simulink model "gm_uz_pmsm_model_9ph_21b_all_double"  (R2021b)
settings: Solver=FixedStepDiscrete  StartTime=0.0  StopTime=0.8  RelTol=1e-3
PreLoadFcn:
  | uz_pmsm_model_9ph_init_parameter
undefined symbols (not defined in the file or in its folder): a, b, c, friction_coefficient, inertia, k_i_d, k_i_q, k_p_d, k_p_q, Kpd, L_d, L_o1, L_o2, L_q, L_x1, L_x2, L_y1, L_y2, L_zero, polepair, psi_pm, R_1, static_friction_torque, Tnd
libraries: hdlmdlgenlib x139, hdlsllib x90, dspsigops x21, simulink x3, slpidlib x2, spsAlphaBetaZerotodq0Lib x1, pid_lib x1, spsdq0toAlphaBetaZeroLib x1
(part 4 of 5)

== system gm_uz_pmsm_model_9ph_21b_all_double/uz_pmsm_model_9ph/Line-Line to Phase voltage2/alpha_beta_0   to   abc ==
  "alpha, beta, 0  " : Inport  OutDataTypeStr=fixdt(1, 25, 12)  PortDimensions=[3]  SampleTime=1e-08
  Gain4_const : Constant  Value=[1;-0.5;-0.5;0;0.86602783203125;-0.86602783203125;1;1;1]  OutDataTypeStr=fixdt(1, 18, 16)  SampleTime=1e-08
  HwModeRegister : Delay  DelayLength=double(1)  InitialCondition=0  SampleTime=1e-08
  HwModeRegister1 : Delay  DelayLength=double(1)  InitialCondition=0  SampleTime=1e-08
  MMul_add_01 : Sum  OutDataTypeStr=fixdt(1, 25, 12)  SaturateOnIntegerOverflow=on  SampleTime=1e-08
  MMul_add_12 : Sum  OutDataTypeStr=fixdt(1, 25, 12)  SaturateOnIntegerOverflow=on  SampleTime=1e-08
  MMul_dot_product : Product  Inputs=**  OutDataTypeStr=fixdt(1, 43, 28)  SampleTime=1e-08
  MMul_dot_product_out_dtc : DataTypeConversion  OutDataTypeStr=fixdt(1, 25, 12)  SampleTime=1e-08  SaturateOnIntegerOverflow=on
  PipelineRegister : Delay  DelayLength=double(1)  InitialCondition=0  SampleTime=1e-08
  Reshape : Reshape  OutputDimensionality=Column vector (2-D)
  Row2Col_in0 : Reshape  OutputDimensionality=Column vector (2-D)
  Row2Col_in1 : Reshape  OutputDimensionality=Column vector (2-D)
  reshape_dotProduct : Reshape  OutputDimensionality=Customize  OutputDimensions=[3,3]
  reshape_mmulResult : Reshape  OutputDimensionality=Customize  OutputDimensions=[3,1]
  select_0 : Selector  NumberOfDimensions=2  SampleTime=1e-08  IndexOptions=Index vector (dialog),Select all  Indices=double(1),[]  OutputSizes=1
  select_1 : Selector  NumberOfDimensions=2  SampleTime=1e-08  IndexOptions=Index vector (dialog),Select all  Indices=double(2),[]  OutputSizes=1
  select_2 : Selector  NumberOfDimensions=2  SampleTime=1e-08  IndexOptions=Index vector (dialog),Select all  Indices=double(3),[]  OutputSizes=1
  select_indices0 : Selector  SampleTime=1e-08  IndexOptions=Index vector (dialog)  Indices=double([1 4 7 2 5 8 3 6 9])  OutputSizes=1
  select_indices1 : Selector  SampleTime=1e-08  IndexOptions=Index vector (dialog)  Indices=double([1 2 3 1 2 3 1 2 3])  OutputSizes=1
  t : Reshape  OutputDimensionality=Customize  OutputDimensions=[3,3]
  vectorized_in0 : Reshape  OutputDimensionality=Row vector (2-D)
  "a, b, c" : Outport  SampleTime=1e-08
  wires:
  reshape_mmulResult/1 -> "a, b, c"/1
  Reshape/1 -> select_indices1/1
  t/1 -> vectorized_in0/1
  vectorized_in0/1 -> select_indices0/1
  select_indices0/1 -> Row2Col_in0/1
  select_indices1/1 -> Row2Col_in1/1
  Row2Col_in0/1 -> HwModeRegister/1
  Row2Col_in1/1 -> HwModeRegister1/1
  MMul_dot_product_out_dtc/1 -> reshape_dotProduct/1
  reshape_dotProduct/1 -> select_2/1, select_1/1, select_0/1
  select_0/1 -> MMul_add_01/1
  select_1/1 -> MMul_add_01/2
  MMul_add_01/1 -> MMul_add_12/1
  select_2/1 -> MMul_add_12/2
  MMul_add_12/1 -> reshape_mmulResult/1
  Gain4_const/1 -> t/1
  PipelineRegister/1 -> MMul_dot_product_out_dtc/1
  "alpha, beta, 0  "/1 -> Reshape/1
  MMul_dot_product/1 -> PipelineRegister/1
  HwModeRegister/1 -> MMul_dot_product/1
  HwModeRegister1/1 -> MMul_dot_product/2

== system gm_uz_pmsm_model_9ph_21b_all_double/uz_pmsm_model_9ph/Transformation/Add ==
  In1 : Inport
  In2 : Inport  Port=2
  Add : Sum  OutDataTypeStr=single  SampleTime=1e-08
  Add_pd1 : Delay  DelayLength=6
  Out1 : Outport
  wires:
  In1/1 -> Add/1
  In2/1 -> Add/2
  Add/1 -> Add_pd1/1
  Add_pd1/1 -> Out1/1

== system gm_uz_pmsm_model_9ph_21b_all_double/uz_pmsm_model_9ph/Transformation/Add1 ==
  In1 : Inport
  In2 : Inport  Port=2
  Add1 : Sum  Inputs=+-  OutDataTypeStr=single  SampleTime=1e-08
  Add1_pd1 : Delay  DelayLength=6
  Out1 : Outport
  wires:
  In1/1 -> Add1/1
  In2/1 -> Add1/2
  Add1/1 -> Add1_pd1/1
  Add1_pd1/1 -> Out1/1

== system gm_uz_pmsm_model_9ph_21b_all_double/uz_pmsm_model_9ph/Transformation/Data Type Conversion39 ==
  In1 : Inport
  Data Type Conversion39 : DataTypeConversion  OutDataTypeStr=single  RndMeth=Nearest  SampleTime=1e-08
  Data Type Conversion39_pd1 : Delay  DelayLength=6
  Out1 : Outport
  wires:
  In1/1 -> Data Type Conversion39/1
  Data Type Conversion39/1 -> Data Type Conversion39_pd1/1
  Data Type Conversion39_pd1/1 -> Out1/1

== system gm_uz_pmsm_model_9ph_21b_all_double/uz_pmsm_model_9ph/Transformation/Divide ==
  In1 : Inport
  In2 : Inport  Port=2
  Divide : Product  Inputs=**  OutDataTypeStr=single  SampleTime=1e-08
  Divide_pd1 : Delay  DelayLength=6
  Out1 : Outport
  wires:
  In1/1 -> Divide/1
  In2/1 -> Divide/2
  Divide/1 -> Divide_pd1/1
  Divide_pd1/1 -> Out1/1

== system gm_uz_pmsm_model_9ph_21b_all_double/uz_pmsm_model_9ph/Transformation/Divide1 ==
  In1 : Inport
  In2 : Inport  Port=2
  Divide1 : Product  Inputs=**  OutDataTypeStr=single  SampleTime=1e-08
  Divide1_pd1 : Delay  DelayLength=6
  Out1 : Outport
  wires:
  In1/1 -> Divide1/1
  In2/1 -> Divide1/2
  Divide1/1 -> Divide1_pd1/1
  Divide1_pd1/1 -> Out1/1

== system gm_uz_pmsm_model_9ph_21b_all_double/uz_pmsm_model_9ph/Transformation/Divide2 ==
  In1 : Inport
  In2 : Inport  Port=2
  Divide2 : Product  Inputs=**  OutDataTypeStr=single  SampleTime=1e-08
  Divide2_pd1 : Delay  DelayLength=6
  Out1 : Outport
  wires:
  In1/1 -> Divide2/1
  In2/1 -> Divide2/2
  Divide2/1 -> Divide2_pd1/1
  Divide2_pd1/1 -> Out1/1

== system gm_uz_pmsm_model_9ph_21b_all_double/uz_pmsm_model_9ph/Transformation/Divide3 ==
  In1 : Inport
  In2 : Inport  Port=2
  Divide3 : Product  Inputs=**  OutDataTypeStr=single  SampleTime=1e-08
  Divide3_pd1 : Delay  DelayLength=6
  Out1 : Outport
  wires:
  In1/1 -> Divide3/1
  In2/1 -> Divide3/2
  Divide3/1 -> Divide3_pd1/1
  Divide3_pd1/1 -> Out1/1

== system gm_uz_pmsm_model_9ph_21b_all_double/uz_pmsm_model_9ph/Transformation/t3 ==
  in0 : Inport
  ColVec1 : Selector  NumberOfDimensions=2  IndexOptions=Select all,Index vector (dialog)  Indices=1,1  OutputSizes=1,1
  ColVec2 : Selector  NumberOfDimensions=2  IndexOptions=Select all,Index vector (dialog)  Indices=1,2  OutputSizes=1,1
  ColVec3 : Selector  NumberOfDimensions=2  IndexOptions=Select all,Index vector (dialog)  Indices=1,3  OutputSizes=1,1
  ColVec4 : Selector  NumberOfDimensions=2  IndexOptions=Select all,Index vector (dialog)  Indices=1,4  OutputSizes=1,1
  ColVec5 : Selector  NumberOfDimensions=2  IndexOptions=Select all,Index vector (dialog)  Indices=1,5  OutputSizes=1,1
  ColVec6 : Selector  NumberOfDimensions=2  IndexOptions=Select all,Index vector (dialog)  Indices=1,6  OutputSizes=1,1
  ColVec7 : Selector  NumberOfDimensions=2  IndexOptions=Select all,Index vector (dialog)  Indices=1,7  OutputSizes=1,1
  ColVec8 : Selector  NumberOfDimensions=2  IndexOptions=Select all,Index vector (dialog)  Indices=1,8  OutputSizes=1,1
  ColVec9 : Selector  NumberOfDimensions=2  IndexOptions=Select all,Index vector (dialog)  Indices=1,9  OutputSizes=1,1
  out0 : Outport
  out1 : Outport  Port=2
  out2 : Outport  Port=3
  out3 : Outport  Port=4
  out4 : Outport  Port=5
  out5 : Outport  Port=6
  out6 : Outport  Port=7
  out7 : Outport  Port=8
  out8 : Outport  Port=9
  wires:
  in0/1 -> ColVec1/1, ColVec2/1, ColVec3/1, ColVec4/1, ColVec5/1, ColVec6/1, ColVec7/1, ColVec8/1, ColVec9/1
  ColVec1/1 -> out0/1
  ColVec2/1 -> out1/1
  ColVec3/1 -> out2/1
  ColVec4/1 -> out3/1
  ColVec5/1 -> out4/1
  ColVec6/1 -> out5/1
  ColVec7/1 -> out6/1
  ColVec8/1 -> out7/1
  ColVec9/1 -> out8/1

== system gm_uz_pmsm_model_9ph_21b_all_double/uz_pmsm_model_9ph/Transformation1/Add ==
  In1 : Inport
  In2 : Inport  Port=2
  Add : Sum  Inputs=+-  OutDataTypeStr=single  SampleTime=1e-08
  Add_pd1 : Delay  DelayLength=6
  Out1 : Outport
  wires:
  In1/1 -> Add/1
  In2/1 -> Add/2
  Add/1 -> Add_pd1/1
  Add_pd1/1 -> Out1/1

== system gm_uz_pmsm_model_9ph_21b_all_double/uz_pmsm_model_9ph/Transformation1/Add1 ==
  In1 : Inport
  In2 : Inport  Port=2
  Add1 : Sum  OutDataTypeStr=single  SampleTime=1e-08
  Add1_pd1 : Delay  DelayLength=6
  Out1 : Outport
  wires:
  In1/1 -> Add1/1
  In2/1 -> Add1/2
  Add1/1 -> Add1_pd1/1
  Add1_pd1/1 -> Out1/1

== system gm_uz_pmsm_model_9ph_21b_all_double/uz_pmsm_model_9ph/Transformation1/Data Type Conversion28 ==
  In1 : Inport
  Data Type Conversion28 : DataTypeConversion  OutDataTypeStr=fixdt(1, 25, 12)  RndMeth=Nearest  SampleTime=1e-08
  Data Type Conversion28_pd1 : Delay  DelayLength=6
  Out1 : Outport
  wires:
  In1/1 -> Data Type Conversion28/1
  Data Type Conversion28/1 -> Data Type Conversion28_pd1/1
  Data Type Conversion28_pd1/1 -> Out1/1

== system gm_uz_pmsm_model_9ph_21b_all_double/uz_pmsm_model_9ph/Transformation1/Divide ==
  In1 : Inport
  In2 : Inport  Port=2
  Divide : Product  Inputs=**  OutDataTypeStr=single  SampleTime=1e-08
  Divide_pd1 : Delay  DelayLength=6
  Out1 : Outport
  wires:
  In1/1 -> Divide/1
  In2/1 -> Divide/2
  Divide/1 -> Divide_pd1/1
  Divide_pd1/1 -> Out1/1

== system gm_uz_pmsm_model_9ph_21b_all_double/uz_pmsm_model_9ph/Transformation1/Divide1 ==
  In1 : Inport
  In2 : Inport  Port=2
  Divide1 : Product  Inputs=**  OutDataTypeStr=single  SampleTime=1e-08
  Divide1_pd1 : Delay  DelayLength=6
  Out1 : Outport
  wires:
  In1/1 -> Divide1/1
  In2/1 -> Divide1/2
  Divide1/1 -> Divide1_pd1/1
  Divide1_pd1/1 -> Out1/1

== system gm_uz_pmsm_model_9ph_21b_all_double/uz_pmsm_model_9ph/Transformation1/Divide2 ==
  In1 : Inport
  In2 : Inport  Port=2
  Divide2 : Product  Inputs=**  OutDataTypeStr=single  SampleTime=1e-08
  Divide2_pd1 : Delay  DelayLength=6
  Out1 : Outport
  wires:
  In1/1 -> Divide2/1
  In2/1 -> Divide2/2
  Divide2/1 -> Divide2_pd1/1
  Divide2_pd1/1 -> Out1/1

== system gm_uz_pmsm_model_9ph_21b_all_double/uz_pmsm_model_9ph/Transformation1/Divide3 ==
  In1 : Inport
  In2 : Inport  Port=2
  Divide3 : Product  Inputs=**  OutDataTypeStr=single  SampleTime=1e-08
  Divide3_pd1 : Delay  DelayLength=6
  Out1 : Outport
  wires:
  In1/1 -> Divide3/1
  In2/1 -> Divide3/2
  Divide3/1 -> Divide3_pd1/1
  Divide3_pd1/1 -> Out1/1

== system gm_uz_pmsm_model_9ph_21b_all_double/uz_pmsm_model_9ph/Transformation1/Transformation1_MAC ==
  in0 : Inport  OutDataTypeStr=fixdt(1, 18, 16)  PortDimensions=[9 1]  SampleTime=1e-08
  in1 : Inport  Port=2  OutDataTypeStr=fixdt(1, 25, 12)  PortDimensions=[9]  SampleTime=1e-08
  globalSchedule : EnablePort  OutDataTypeStr=boolean
  PipelineRegister : Delay  DelayLength=double(8)  InitialCondition=0
  t : hdlsllib/HDL Operations/Multiply-Accumulate  opMode=Vector  initValueSetting=Dialog  initValue=0  initValueSetting2=Dialog  initValue2=0  initValueSetting3=Dialog  initValue3=0  num_samples=2  RndMeth2=Floor  RndMeth3=Floor  OutDataTypeStr=fixdt(1, 25, 12)  datatype2=Inherit: Inherit via back propagation  datatype3=Inherit: Inherit via back propagation  validOut=on  endInandOut=on  startOut=on  countOut=on  dim=-1  DoSatur=off  parallel=off
      settings: SourceProductBaseCode=SL
  out0 : Outport  OutDataTypeStr=fixdt(1, 25, 12)  SampleTime=1e-08  InitialOutput=0
  wires:
  PipelineRegister/1 -> out0/1
  in0/1 -> t/1
  in1/1 -> t/2
  t/1 -> PipelineRegister/1

== system gm_uz_pmsm_model_9ph_21b_all_double/uz_pmsm_model_9ph/Transformation1/Transformation1_MAC1 ==
  in0 : Inport  OutDataTypeStr=fixdt(1, 18, 16)  PortDimensions=[9 1]  SampleTime=1e-08
  in1 : Inport  Port=2  OutDataTypeStr=fixdt(1, 25, 12)  PortDimensions=[9]  SampleTime=1e-08
  globalSchedule : EnablePort  OutDataTypeStr=boolean
  PipelineRegister : Delay  DelayLength=double(8)  InitialCondition=0
  t : hdlsllib/HDL Operations/Multiply-Accumulate  opMode=Vector  initValueSetting=Dialog  initValue=0  initValueSetting2=Dialog  initValue2=0  initValueSetting3=Dialog  initValue3=0  num_samples=2  RndMeth2=Floor  RndMeth3=Floor  OutDataTypeStr=fixdt(1, 25, 12)  datatype2=Inherit: Inherit via back propagation  datatype3=Inherit: Inherit via back propagation  validOut=on  endInandOut=on  startOut=on  countOut=on  dim=-1  DoSatur=off  parallel=off
      settings: SourceProductBaseCode=SL
  out0 : Outport  OutDataTypeStr=fixdt(1, 25, 12)  SampleTime=1e-08  InitialOutput=0
  wires:
  PipelineRegister/1 -> out0/1
  in0/1 -> t/1
  in1/1 -> t/2
  t/1 -> PipelineRegister/1

== system gm_uz_pmsm_model_9ph_21b_all_double/uz_pmsm_model_9ph/Transformation1/Transformation1_MAC2 ==
  in0 : Inport  OutDataTypeStr=fixdt(1, 18, 16)  PortDimensions=[9 1]  SampleTime=1e-08
  in1 : Inport  Port=2  OutDataTypeStr=fixdt(1, 25, 12)  PortDimensions=[9]  SampleTime=1e-08
  globalSchedule : EnablePort  OutDataTypeStr=boolean
  PipelineRegister : Delay  DelayLength=double(8)  InitialCondition=0
  t : hdlsllib/HDL Operations/Multiply-Accumulate  opMode=Vector  initValueSetting=Dialog  initValue=0  initValueSetting2=Dialog  initValue2=0  initValueSetting3=Dialog  initValue3=0  num_samples=2  RndMeth2=Floor  RndMeth3=Floor  OutDataTypeStr=fixdt(1, 25, 12)  datatype2=Inherit: Inherit via back propagation  datatype3=Inherit: Inherit via back propagation  validOut=on  endInandOut=on  startOut=on  countOut=on  dim=-1  DoSatur=off  parallel=off
      settings: SourceProductBaseCode=SL
  out0 : Outport  OutDataTypeStr=fixdt(1, 25, 12)  SampleTime=1e-08  InitialOutput=0
  wires:
  PipelineRegister/1 -> out0/1
  in0/1 -> t/1
  in1/1 -> t/2
  t/1 -> PipelineRegister/1

== system gm_uz_pmsm_model_9ph_21b_all_double/uz_pmsm_model_9ph/Transformation1/Transformation1_MAC3 ==
  in0 : Inport  OutDataTypeStr=fixdt(1, 18, 16)  PortDimensions=[9 1]  SampleTime=1e-08
  in1 : Inport  Port=2  OutDataTypeStr=fixdt(1, 25, 12)  PortDimensions=[9]  SampleTime=1e-08
  globalSchedule : EnablePort  OutDataTypeStr=boolean
  PipelineRegister : Delay  DelayLength=double(8)  InitialCondition=0
  t : hdlsllib/HDL Operations/Multiply-Accumulate  opMode=Vector  initValueSetting=Dialog  initValue=0  initValueSetting2=Dialog  initValue2=0  initValueSetting3=Dialog  initValue3=0  num_samples=2  RndMeth2=Floor  RndMeth3=Floor  OutDataTypeStr=fixdt(1, 25, 12)  datatype2=Inherit: Inherit via back propagation  datatype3=Inherit: Inherit via back propagation  validOut=on  endInandOut=on  startOut=on  countOut=on  dim=-1  DoSatur=off  parallel=off
      settings: SourceProductBaseCode=SL
  out0 : Outport  OutDataTypeStr=fixdt(1, 25, 12)  SampleTime=1e-08  InitialOutput=0
  wires:
  PipelineRegister/1 -> out0/1
  in0/1 -> t/1
  in1/1 -> t/2
  t/1 -> PipelineRegister/1

== system gm_uz_pmsm_model_9ph_21b_all_double/uz_pmsm_model_9ph/Transformation1/Transformation1_MAC4 ==
  in0 : Inport  OutDataTypeStr=fixdt(1, 18, 16)  PortDimensions=[9 1]  SampleTime=1e-08
  in1 : Inport  Port=2  OutDataTypeStr=fixdt(1, 25, 12)  PortDimensions=[9]  SampleTime=1e-08
  globalSchedule : EnablePort  OutDataTypeStr=boolean
  PipelineRegister : Delay  DelayLength=double(8)  InitialCondition=0
  t : hdlsllib/HDL Operations/Multiply-Accumulate  opMode=Vector  initValueSetting=Dialog  initValue=0  initValueSetting2=Dialog  initValue2=0  initValueSetting3=Dialog  initValue3=0  num_samples=2  RndMeth2=Floor  RndMeth3=Floor  OutDataTypeStr=fixdt(1, 25, 12)  datatype2=Inherit: Inherit via back propagation  datatype3=Inherit: Inherit via back propagation  validOut=on  endInandOut=on  startOut=on  countOut=on  dim=-1  DoSatur=off  parallel=off
      settings: SourceProductBaseCode=SL
  out0 : Outport  OutDataTypeStr=fixdt(1, 25, 12)  SampleTime=1e-08  InitialOutput=0
  wires:
  PipelineRegister/1 -> out0/1
  in0/1 -> t/1
  in1/1 -> t/2
  t/1 -> PipelineRegister/1

== system gm_uz_pmsm_model_9ph_21b_all_double/uz_pmsm_model_9ph/Transformation1/Transformation1_MAC5 ==
  in0 : Inport  OutDataTypeStr=fixdt(1, 18, 16)  PortDimensions=[9 1]  SampleTime=1e-08
  in1 : Inport  Port=2  OutDataTypeStr=fixdt(1, 25, 12)  PortDimensions=[9]  SampleTime=1e-08
  globalSchedule : EnablePort  OutDataTypeStr=boolean
  PipelineRegister : Delay  DelayLength=double(8)  InitialCondition=0
  t : hdlsllib/HDL Operations/Multiply-Accumulate  opMode=Vector  initValueSetting=Dialog  initValue=0  initValueSetting2=Dialog  initValue2=0  initValueSetting3=Dialog  initValue3=0  num_samples=2  RndMeth2=Floor  RndMeth3=Floor  OutDataTypeStr=fixdt(1, 25, 12)  datatype2=Inherit: Inherit via back propagation  datatype3=Inherit: Inherit via back propagation  validOut=on  endInandOut=on  startOut=on  countOut=on  dim=-1  DoSatur=off  parallel=off
      settings: SourceProductBaseCode=SL
  out0 : Outport  OutDataTypeStr=fixdt(1, 25, 12)  SampleTime=1e-08  InitialOutput=0
  wires:
  PipelineRegister/1 -> out0/1
  in0/1 -> t/1
  in1/1 -> t/2
  t/1 -> PipelineRegister/1

== system gm_uz_pmsm_model_9ph_21b_all_double/uz_pmsm_model_9ph/Transformation1/Transformation1_MAC6 ==
  in0 : Inport  OutDataTypeStr=fixdt(1, 18, 16)  PortDimensions=[9 1]  SampleTime=1e-08
  in1 : Inport  Port=2  OutDataTypeStr=fixdt(1, 25, 12)  PortDimensions=[9]  SampleTime=1e-08
  globalSchedule : EnablePort  OutDataTypeStr=boolean
  PipelineRegister : Delay  DelayLength=double(8)  InitialCondition=0
  t : hdlsllib/HDL Operations/Multiply-Accumulate  opMode=Vector  initValueSetting=Dialog  initValue=0  initValueSetting2=Dialog  initValue2=0  initValueSetting3=Dialog  initValue3=0  num_samples=2  RndMeth2=Floor  RndMeth3=Floor  OutDataTypeStr=fixdt(1, 25, 12)  datatype2=Inherit: Inherit via back propagation  datatype3=Inherit: Inherit via back propagation  validOut=on  endInandOut=on  startOut=on  countOut=on  dim=-1  DoSatur=off  parallel=off
      settings: SourceProductBaseCode=SL
  out0 : Outport  OutDataTypeStr=fixdt(1, 25, 12)  SampleTime=1e-08  InitialOutput=0
  wires:
  PipelineRegister/1 -> out0/1
  in0/1 -> t/1
  in1/1 -> t/2
  t/1 -> PipelineRegister/1

== system gm_uz_pmsm_model_9ph_21b_all_double/uz_pmsm_model_9ph/Transformation1/Transformation1_MAC7 ==
  in0 : Inport  OutDataTypeStr=fixdt(1, 18, 16)  PortDimensions=[9 1]  SampleTime=1e-08
  in1 : Inport  Port=2  OutDataTypeStr=fixdt(1, 25, 12)  PortDimensions=[9]  SampleTime=1e-08
  globalSchedule : EnablePort  OutDataTypeStr=boolean
  PipelineRegister : Delay  DelayLength=double(8)  InitialCondition=0
  t : hdlsllib/HDL Operations/Multiply-Accumulate  opMode=Vector  initValueSetting=Dialog  initValue=0  initValueSetting2=Dialog  initValue2=0  initValueSetting3=Dialog  initValue3=0  num_samples=2  RndMeth2=Floor  RndMeth3=Floor  OutDataTypeStr=fixdt(1, 25, 12)  datatype2=Inherit: Inherit via back propagation  datatype3=Inherit: Inherit via back propagation  validOut=on  endInandOut=on  startOut=on  countOut=on  dim=-1  DoSatur=off  parallel=off
      settings: SourceProductBaseCode=SL
  out0 : Outport  OutDataTypeStr=fixdt(1, 25, 12)  SampleTime=1e-08  InitialOutput=0
  wires:
  PipelineRegister/1 -> out0/1
  in0/1 -> t/1
  in1/1 -> t/2
  t/1 -> PipelineRegister/1

== system gm_uz_pmsm_model_9ph_21b_all_double/uz_pmsm_model_9ph/Transformation1/Transformation1_MAC8 ==
  in0 : Inport  OutDataTypeStr=fixdt(1, 18, 16)  PortDimensions=[9 1]  SampleTime=1e-08
  in1 : Inport  Port=2  OutDataTypeStr=fixdt(1, 25, 12)  PortDimensions=[9]  SampleTime=1e-08
  globalSchedule : EnablePort  OutDataTypeStr=boolean
  PipelineRegister : Delay  DelayLength=double(8)  InitialCondition=0
  t : hdlsllib/HDL Operations/Multiply-Accumulate  opMode=Vector  initValueSetting=Dialog  initValue=0  initValueSetting2=Dialog  initValue2=0  initValueSetting3=Dialog  initValue3=0  num_samples=2  RndMeth2=Floor  RndMeth3=Floor  OutDataTypeStr=fixdt(1, 25, 12)  datatype2=Inherit: Inherit via back propagation  datatype3=Inherit: Inherit via back propagation  validOut=on  endInandOut=on  startOut=on  countOut=on  dim=-1  DoSatur=off  parallel=off
      settings: SourceProductBaseCode=SL
  out0 : Outport  OutDataTypeStr=fixdt(1, 25, 12)  SampleTime=1e-08  InitialOutput=0
  wires:
  PipelineRegister/1 -> out0/1
  in0/1 -> t/1
  in1/1 -> t/2
  t/1 -> PipelineRegister/1

== system gm_uz_pmsm_model_9ph_21b_all_double/uz_pmsm_model_9ph/Transformation1/t3 ==
  in0 : Inport
  ColVec1 : Selector  NumberOfDimensions=2  IndexOptions=Select all,Index vector (dialog)  Indices=1,1  OutputSizes=1,1
  ColVec2 : Selector  NumberOfDimensions=2  IndexOptions=Select all,Index vector (dialog)  Indices=1,2  OutputSizes=1,1
  ColVec3 : Selector  NumberOfDimensions=2  IndexOptions=Select all,Index vector (dialog)  Indices=1,3  OutputSizes=1,1
  ColVec4 : Selector  NumberOfDimensions=2  IndexOptions=Select all,Index vector (dialog)  Indices=1,4  OutputSizes=1,1
  ColVec5 : Selector  NumberOfDimensions=2  IndexOptions=Select all,Index vector (dialog)  Indices=1,5  OutputSizes=1,1
  ColVec6 : Selector  NumberOfDimensions=2  IndexOptions=Select all,Index vector (dialog)  Indices=1,6  OutputSizes=1,1
  ColVec7 : Selector  NumberOfDimensions=2  IndexOptions=Select all,Index vector (dialog)  Indices=1,7  OutputSizes=1,1
  ColVec8 : Selector  NumberOfDimensions=2  IndexOptions=Select all,Index vector (dialog)  Indices=1,8  OutputSizes=1,1
  ColVec9 : Selector  NumberOfDimensions=2  IndexOptions=Select all,Index vector (dialog)  Indices=1,9  OutputSizes=1,1
  out0 : Outport
  out1 : Outport  Port=2
  out2 : Outport  Port=3
  out3 : Outport  Port=4
  out4 : Outport  Port=5
  out5 : Outport  Port=6
  out6 : Outport  Port=7
  out7 : Outport  Port=8
  out8 : Outport  Port=9
  wires:
  in0/1 -> ColVec1/1, ColVec2/1, ColVec3/1, ColVec4/1, ColVec5/1, ColVec6/1, ColVec7/1, ColVec8/1, ColVec9/1
  ColVec1/1 -> out0/1
  ColVec2/1 -> out1/1
  ColVec3/1 -> out2/1
  ColVec4/1 -> out3/1
  ColVec5/1 -> out4/1
  ColVec6/1 -> out5/1
  ColVec7/1 -> out6/1
  ColVec8/1 -> out7/1
  ColVec9/1 -> out8/1

== system gm_uz_pmsm_model_9ph_21b_all_double/uz_pmsm_model_9ph/dq_model_9ph/Add ==
  In1 : Inport
  In2 : Inport  Port=2
  Add : Sum  Inputs=+-  OutDataTypeStr=double  SampleTime=1e-08
  Add_pd1 : Delay  DelayLength=6
  Out1 : Outport
  wires:
  In1/1 -> Add/1
  In2/1 -> Add/2
  Add/1 -> Add_pd1/1
  Add_pd1/1 -> Out1/1

== system gm_uz_pmsm_model_9ph_21b_all_double/uz_pmsm_model_9ph/dq_model_9ph/Add1 ==
  In1 : Inport
  In2 : Inport  Port=2
  Add1 : Sum  Inputs=+-  OutDataTypeStr=double  SampleTime=1e-08
  Add1_pd1 : Delay  DelayLength=6
  Out1 : Outport
  wires:
  In1/1 -> Add1/1
  In2/1 -> Add1/2
  Add1/1 -> Add1_pd1/1
  Add1_pd1/1 -> Out1/1

== system gm_uz_pmsm_model_9ph_21b_all_double/uz_pmsm_model_9ph/dq_model_9ph/Add2 ==
  In1 : Inport
  In2 : Inport  Port=2
  Add2 : Sum  Inputs=+-  OutDataTypeStr=double  SampleTime=1e-08
  Add2_pd1 : Delay  DelayLength=6
  Out1 : Outport
  wires:
  In1/1 -> Add2/1
  In2/1 -> Add2/2
  Add2/1 -> Add2_pd1/1
  Add2_pd1/1 -> Out1/1

== system gm_uz_pmsm_model_9ph_21b_all_double/uz_pmsm_model_9ph/dq_model_9ph/Add3 ==
  In1 : Inport
  In2 : Inport  Port=2
  Add3 : Sum  Inputs=+-  OutDataTypeStr=double  SampleTime=1e-08
  Add3_pd1 : Delay  DelayLength=6
  Out1 : Outport
  wires:
  In1/1 -> Add3/1
  In2/1 -> Add3/2
  Add3/1 -> Add3_pd1/1
  Add3_pd1/1 -> Out1/1

== system gm_uz_pmsm_model_9ph_21b_all_double/uz_pmsm_model_9ph/dq_model_9ph/Add4 ==
  In1 : Inport
  In2 : Inport  Port=2
  Add4 : Sum  Inputs=+-  OutDataTypeStr=double  SampleTime=1e-08
  Add4_pd1 : Delay  DelayLength=6
  Out1 : Outport
  wires:
  In1/1 -> Add4/1
  In2/1 -> Add4/2
  Add4/1 -> Add4_pd1/1
  Add4_pd1/1 -> Out1/1

== system gm_uz_pmsm_model_9ph_21b_all_double/uz_pmsm_model_9ph/dq_model_9ph/Add5 ==
  In1 : Inport
  In2 : Inport  Port=2
  Add5 : Sum  Inputs=+-  OutDataTypeStr=double  SampleTime=1e-08
  Add5_pd1 : Delay  DelayLength=6
  Out1 : Outport
  wires:
  In1/1 -> Add5/1
  In2/1 -> Add5/2
  Add5/1 -> Add5_pd1/1
  Add5_pd1/1 -> Out1/1

== system gm_uz_pmsm_model_9ph_21b_all_double/uz_pmsm_model_9ph/dq_model_9ph/Add6 ==
  In1 : Inport
  In2 : Inport  Port=2
  Add6 : Sum  Inputs=+-  OutDataTypeStr=double  SampleTime=1e-08
  Add6_pd1 : Delay  DelayLength=6
  Out1 : Outport
  wires:
  In1/1 -> Add6/1
  In2/1 -> Add6/2
  Add6/1 -> Add6_pd1/1
  Add6_pd1/1 -> Out1/1

== system gm_uz_pmsm_model_9ph_21b_all_double/uz_pmsm_model_9ph/dq_model_9ph/Compare To Constant1_relop ==
  In1 : Inport
  In2 : Inport  Port=2
  Compare To Constant1_relop : RelationalOperator  Operator=<  OutDataTypeStr=boolean  SampleTime=1e-08  RndMeth=Nearest  InputSameDT=on
  Compare To Constant1_relop_pd1 : Delay  DelayLength=1
  Out1 : Outport
  wires:
  In1/1 -> Compare To Constant1_relop/1
  In2/1 -> Compare To Constant1_relop/2
  Compare To Constant1_relop/1 -> Compare To Constant1_relop_pd1/1
  Compare To Constant1_relop_pd1/1 -> Out1/1

== system gm_uz_pmsm_model_9ph_21b_all_double/uz_pmsm_model_9ph/dq_model_9ph/Compare To Constant_relop ==
  In1 : Inport
  In2 : Inport  Port=2
  Compare To Constant_relop : RelationalOperator  OutDataTypeStr=boolean  SampleTime=1e-08  RndMeth=Nearest  InputSameDT=on
  Compare To Constant_relop_pd1 : Delay  DelayLength=1
  Out1 : Outport
  wires:
  In1/1 -> Compare To Constant_relop/1
  In2/1 -> Compare To Constant_relop/2
  Compare To Constant_relop/1 -> Compare To Constant_relop_pd1/1
  Compare To Constant_relop_pd1/1 -> Out1/1

== system gm_uz_pmsm_model_9ph_21b_all_double/uz_pmsm_model_9ph/dq_model_9ph/Data Type Conversion ==
  In1 : Inport
  Data Type Conversion : DataTypeConversion  OutDataTypeStr=double  RndMeth=Nearest  SampleTime=1e-08
  Data Type Conversion_pd1 : Delay  DelayLength=3
  Out1 : Outport
  wires:
  In1/1 -> Data Type Conversion/1
  Data Type Conversion/1 -> Data Type Conversion_pd1/1
  Data Type Conversion_pd1/1 -> Out1/1

== system gm_uz_pmsm_model_9ph_21b_all_double/uz_pmsm_model_9ph/dq_model_9ph/Data Type Conversion1 ==
  In1 : Inport
  Data Type Conversion1 : DataTypeConversion  OutDataTypeStr=double  RndMeth=Nearest  SampleTime=1e-08
  Data Type Conversion1_pd1 : Delay  DelayLength=3
  Out1 : Outport
  wires:
  In1/1 -> Data Type Conversion1/1
  Data Type Conversion1/1 -> Data Type Conversion1_pd1/1
  Data Type Conversion1_pd1/1 -> Out1/1

== system gm_uz_pmsm_model_9ph_21b_all_double/uz_pmsm_model_9ph/dq_model_9ph/Data Type Conversion10 ==
  In1 : Inport
  Data Type Conversion10 : DataTypeConversion  OutDataTypeStr=double  RndMeth=Nearest  SampleTime=1e-08
  Data Type Conversion10_pd1 : Delay  DelayLength=3
  Out1 : Outport
  wires:
  In1/1 -> Data Type Conversion10/1
  Data Type Conversion10/1 -> Data Type Conversion10_pd1/1
  Data Type Conversion10_pd1/1 -> Out1/1

== system gm_uz_pmsm_model_9ph_21b_all_double/uz_pmsm_model_9ph/dq_model_9ph/Data Type Conversion11 ==
  In1 : Inport
  Data Type Conversion11 : DataTypeConversion  OutDataTypeStr=double  RndMeth=Nearest  SampleTime=1e-08
  Data Type Conversion11_pd1 : Delay  DelayLength=3
  Out1 : Outport
  wires:
  In1/1 -> Data Type Conversion11/1
  Data Type Conversion11/1 -> Data Type Conversion11_pd1/1
  Data Type Conversion11_pd1/1 -> Out1/1

== system gm_uz_pmsm_model_9ph_21b_all_double/uz_pmsm_model_9ph/dq_model_9ph/Data Type Conversion12 ==
  In1 : Inport
  Data Type Conversion12 : DataTypeConversion  OutDataTypeStr=double  RndMeth=Nearest  SampleTime=1e-08
  Data Type Conversion12_pd1 : Delay  DelayLength=3
  Out1 : Outport
  wires:
  In1/1 -> Data Type Conversion12/1
  Data Type Conversion12/1 -> Data Type Conversion12_pd1/1
  Data Type Conversion12_pd1/1 -> Out1/1

== system gm_uz_pmsm_model_9ph_21b_all_double/uz_pmsm_model_9ph/dq_model_9ph/Data Type Conversion13 ==
  In1 : Inport
  Data Type Conversion13 : DataTypeConversion  OutDataTypeStr=double  RndMeth=Nearest  SampleTime=1e-08
  Data Type Conversion13_pd1 : Delay  DelayLength=3
  Out1 : Outport
  wires:
  In1/1 -> Data Type Conversion13/1
  Data Type Conversion13/1 -> Data Type Conversion13_pd1/1
  Data Type Conversion13_pd1/1 -> Out1/1

== system gm_uz_pmsm_model_9ph_21b_all_double/uz_pmsm_model_9ph/dq_model_9ph/Data Type Conversion2 ==
  In1 : Inport
  Data Type Conversion2 : DataTypeConversion  OutDataTypeStr=double  RndMeth=Nearest  SampleTime=1e-08
  Data Type Conversion2_pd1 : Delay  DelayLength=3
  Out1 : Outport
  wires:
  In1/1 -> Data Type Conversion2/1
  Data Type Conversion2/1 -> Data Type Conversion2_pd1/1
  Data Type Conversion2_pd1/1 -> Out1/1

== system gm_uz_pmsm_model_9ph_21b_all_double/uz_pmsm_model_9ph/dq_model_9ph/Data Type Conversion21 ==
  In1 : Inport
  Data Type Conversion21 : DataTypeConversion  OutDataTypeStr=double  RndMeth=Nearest  SampleTime=1e-08
  Data Type Conversion21_pd1 : Delay  DelayLength=3
  Out1 : Outport
  wires:
  In1/1 -> Data Type Conversion21/1
  Data Type Conversion21/1 -> Data Type Conversion21_pd1/1
  Data Type Conversion21_pd1/1 -> Out1/1

== system gm_uz_pmsm_model_9ph_21b_all_double/uz_pmsm_model_9ph/dq_model_9ph/Data Type Conversion3 ==
  In1 : Inport
  Data Type Conversion3 : DataTypeConversion  OutDataTypeStr=single  RndMeth=Nearest  SampleTime=1e-08
  Data Type Conversion3_pd1 : Delay  DelayLength=3
  Out1 : Outport
  wires:
  In1/1 -> Data Type Conversion3/1
  Data Type Conversion3/1 -> Data Type Conversion3_pd1/1
  Data Type Conversion3_pd1/1 -> Out1/1

== system gm_uz_pmsm_model_9ph_21b_all_double/uz_pmsm_model_9ph/dq_model_9ph/Data Type Conversion31 ==
  In1 : Inport
  Data Type Conversion31 : DataTypeConversion  OutDataTypeStr=double  RndMeth=Nearest  SampleTime=1e-08
  Data Type Conversion31_pd1 : Delay  DelayLength=3
  Out1 : Outport
  wires:
  In1/1 -> Data Type Conversion31/1
  Data Type Conversion31/1 -> Data Type Conversion31_pd1/1
  Data Type Conversion31_pd1/1 -> Out1/1

== system gm_uz_pmsm_model_9ph_21b_all_double/uz_pmsm_model_9ph/dq_model_9ph/Data Type Conversion4 ==
  In1 : Inport
  Data Type Conversion4 : DataTypeConversion  OutDataTypeStr=single  RndMeth=Nearest  SampleTime=1e-08
  Data Type Conversion4_pd1 : Delay  DelayLength=3
  Out1 : Outport
  wires:
  In1/1 -> Data Type Conversion4/1
  Data Type Conversion4/1 -> Data Type Conversion4_pd1/1
  Data Type Conversion4_pd1/1 -> Out1/1

== system gm_uz_pmsm_model_9ph_21b_all_double/uz_pmsm_model_9ph/dq_model_9ph/Data Type Conversion41 ==
  In1 : Inport
  Data Type Conversion41 : DataTypeConversion  OutDataTypeStr=double  RndMeth=Nearest  SampleTime=1e-08
  Data Type Conversion41_pd1 : Delay  DelayLength=3
  Out1 : Outport
  wires:
  In1/1 -> Data Type Conversion41/1
  Data Type Conversion41/1 -> Data Type Conversion41_pd1/1
  Data Type Conversion41_pd1/1 -> Out1/1

== system gm_uz_pmsm_model_9ph_21b_all_double/uz_pmsm_model_9ph/dq_model_9ph/Data Type Conversion5 ==
  In1 : Inport
  Data Type Conversion5 : DataTypeConversion  OutDataTypeStr=single  RndMeth=Nearest  SampleTime=1e-08
  Data Type Conversion5_pd1 : Delay  DelayLength=3
  Out1 : Outport
  wires:
  In1/1 -> Data Type Conversion5/1
  Data Type Conversion5/1 -> Data Type Conversion5_pd1/1
  Data Type Conversion5_pd1/1 -> Out1/1

== system gm_uz_pmsm_model_9ph_21b_all_double/uz_pmsm_model_9ph/dq_model_9ph/Data Type Conversion51 ==
  In1 : Inport
  Data Type Conversion51 : DataTypeConversion  OutDataTypeStr=double  RndMeth=Nearest  SampleTime=1e-08
  Data Type Conversion51_pd1 : Delay  DelayLength=3
  Out1 : Outport
  wires:
  In1/1 -> Data Type Conversion51/1
  Data Type Conversion51/1 -> Data Type Conversion51_pd1/1
  Data Type Conversion51_pd1/1 -> Out1/1

== system gm_uz_pmsm_model_9ph_21b_all_double/uz_pmsm_model_9ph/dq_model_9ph/Data Type Conversion6 ==
  In1 : Inport
  Data Type Conversion6 : DataTypeConversion  OutDataTypeStr=single  RndMeth=Nearest  SampleTime=1e-08
  Data Type Conversion6_pd1 : Delay  DelayLength=3
  Out1 : Outport
  wires:
  In1/1 -> Data Type Conversion6/1
  Data Type Conversion6/1 -> Data Type Conversion6_pd1/1
  Data Type Conversion6_pd1/1 -> Out1/1

== system gm_uz_pmsm_model_9ph_21b_all_double/uz_pmsm_model_9ph/dq_model_9ph/Data Type Conversion61 ==
  In1 : Inport
  Data Type Conversion61 : DataTypeConversion  OutDataTypeStr=double  RndMeth=Nearest  SampleTime=1e-08
  Data Type Conversion61_pd1 : Delay  DelayLength=3
  Out1 : Outport
  wires:
  In1/1 -> Data Type Conversion61/1
  Data Type Conversion61/1 -> Data Type Conversion61_pd1/1
  Data Type Conversion61_pd1/1 -> Out1/1

== system gm_uz_pmsm_model_9ph_21b_all_double/uz_pmsm_model_9ph/dq_model_9ph/Data Type Conversion7 ==
  In1 : Inport
  Data Type Conversion7 : DataTypeConversion  OutDataTypeStr=double  RndMeth=Nearest  SampleTime=1e-08
  Data Type Conversion7_pd1 : Delay  DelayLength=3
  Out1 : Outport
  wires:
  In1/1 -> Data Type Conversion7/1
  Data Type Conversion7/1 -> Data Type Conversion7_pd1/1
  Data Type Conversion7_pd1/1 -> Out1/1

== system gm_uz_pmsm_model_9ph_21b_all_double/uz_pmsm_model_9ph/dq_model_9ph/Data Type Conversion71 ==
  In1 : Inport
  Data Type Conversion71 : DataTypeConversion  OutDataTypeStr=double  RndMeth=Nearest  SampleTime=1e-08
  Data Type Conversion71_pd1 : Delay  DelayLength=3
  Out1 : Outport
  wires:
  In1/1 -> Data Type Conversion71/1
  Data Type Conversion71/1 -> Data Type Conversion71_pd1/1
  Data Type Conversion71_pd1/1 -> Out1/1

== system gm_uz_pmsm_model_9ph_21b_all_double/uz_pmsm_model_9ph/dq_model_9ph/Data Type Conversion8 ==
  In1 : Inport
  Data Type Conversion8 : DataTypeConversion  OutDataTypeStr=double  RndMeth=Nearest  SampleTime=1e-08
  Data Type Conversion8_pd1 : Delay  DelayLength=3
  Out1 : Outport
  wires:
  In1/1 -> Data Type Conversion8/1
  Data Type Conversion8/1 -> Data Type Conversion8_pd1/1
  Data Type Conversion8_pd1/1 -> Out1/1

== system gm_uz_pmsm_model_9ph_21b_all_double/uz_pmsm_model_9ph/dq_model_9ph/Data Type Conversion9 ==
  In1 : Inport
  Data Type Conversion9 : DataTypeConversion  OutDataTypeStr=double  RndMeth=Nearest  SampleTime=1e-08
  Data Type Conversion9_pd1 : Delay  DelayLength=3
  Out1 : Outport
  wires:
  In1/1 -> Data Type Conversion9/1
  Data Type Conversion9/1 -> Data Type Conversion9_pd1/1
  Data Type Conversion9_pd1/1 -> Out1/1

== system gm_uz_pmsm_model_9ph_21b_all_double/uz_pmsm_model_9ph/dq_model_9ph/Divide ==
  In1 : Inport
  In2 : Inport  Port=2
  Divide : Product  Inputs=**  OutDataTypeStr=double  SampleTime=1e-08
  Divide_pd1 : Delay  DelayLength=6
  Out1 : Outport
  wires:
  In1/1 -> Divide/1
  In2/1 -> Divide/2
  Divide/1 -> Divide_pd1/1
  Divide_pd1/1 -> Out1/1

== system gm_uz_pmsm_model_9ph_21b_all_double/uz_pmsm_model_9ph/dq_model_9ph/Divide1 ==
  In1 : Inport
  In2 : Inport  Port=2
  Divide1 : Product  Inputs=**  OutDataTypeStr=double  SampleTime=1e-08
  Divide1_pd1 : Delay  DelayLength=6
  Out1 : Outport
  wires:
  In1/1 -> Divide1/1
  In2/1 -> Divide1/2
  Divide1/1 -> Divide1_pd1/1
  Divide1_pd1/1 -> Out1/1

== system gm_uz_pmsm_model_9ph_21b_all_double/uz_pmsm_model_9ph/dq_model_9ph/Divide10 ==
  In1 : Inport
  In2 : Inport  Port=2
  Divide10 : Product  Inputs=**  OutDataTypeStr=double  SampleTime=1e-08
  Divide10_pd1 : Delay  DelayLength=6
  Out1 : Outport
  wires:
  In1/1 -> Divide10/1
  In2/1 -> Divide10/2
  Divide10/1 -> Divide10_pd1/1
  Divide10_pd1/1 -> Out1/1

== system gm_uz_pmsm_model_9ph_21b_all_double/uz_pmsm_model_9ph/dq_model_9ph/Divide11 ==
  In1 : Inport
  In2 : Inport  Port=2
  Divide11 : Product  Inputs=**  OutDataTypeStr=double  SampleTime=1e-08
  Divide11_pd1 : Delay  DelayLength=6
  Out1 : Outport
  wires:
  In1/1 -> Divide11/1
  In2/1 -> Divide11/2
  Divide11/1 -> Divide11_pd1/1
  Divide11_pd1/1 -> Out1/1

== system gm_uz_pmsm_model_9ph_21b_all_double/uz_pmsm_model_9ph/dq_model_9ph/Divide12 ==
  In1 : Inport
  In2 : Inport  Port=2
  Divide12 : Product  Inputs=**  OutDataTypeStr=double  SampleTime=1e-08
  Divide12_pd1 : Delay  DelayLength=6
  Out1 : Outport
  wires:
  In1/1 -> Divide12/1
  In2/1 -> Divide12/2
  Divide12/1 -> Divide12_pd1/1
  Divide12_pd1/1 -> Out1/1

== system gm_uz_pmsm_model_9ph_21b_all_double/uz_pmsm_model_9ph/dq_model_9ph/Divide13 ==
  In1 : Inport
  In2 : Inport  Port=2
  Divide13 : Product  Inputs=**  OutDataTypeStr=double  SampleTime=1e-08
  Divide13_pd1 : Delay  DelayLength=6
  Out1 : Outport
  wires:
  In1/1 -> Divide13/1
  In2/1 -> Divide13/2
  Divide13/1 -> Divide13_pd1/1
  Divide13_pd1/1 -> Out1/1

== system gm_uz_pmsm_model_9ph_21b_all_double/uz_pmsm_model_9ph/dq_model_9ph/Divide2 ==
  In1 : Inport
  In2 : Inport  Port=2
  Divide2 : Product  Inputs=**  OutDataTypeStr=double  SampleTime=1e-08
  Divide2_pd1 : Delay  DelayLength=6
  Out1 : Outport
  wires:
  In1/1 -> Divide2/1
  In2/1 -> Divide2/2
  Divide2/1 -> Divide2_pd1/1
  Divide2_pd1/1 -> Out1/1

== system gm_uz_pmsm_model_9ph_21b_all_double/uz_pmsm_model_9ph/dq_model_9ph/Divide3 ==
  In1 : Inport
  In2 : Inport  Port=2
  Divide3 : Product  Inputs=**  OutDataTypeStr=double  SampleTime=1e-08
  Divide3_pd1 : Delay  DelayLength=6
  Out1 : Outport
  wires:
  In1/1 -> Divide3/1
  In2/1 -> Divide3/2
  Divide3/1 -> Divide3_pd1/1
  Divide3_pd1/1 -> Out1/1

== system gm_uz_pmsm_model_9ph_21b_all_double/uz_pmsm_model_9ph/dq_model_9ph/Divide4 ==
  In1 : Inport
  In2 : Inport  Port=2
  Divide4 : Product  Inputs=**  OutDataTypeStr=double  SampleTime=1e-08
  Divide4_pd1 : Delay  DelayLength=6
  Out1 : Outport
  wires:
  In1/1 -> Divide4/1
  In2/1 -> Divide4/2
  Divide4/1 -> Divide4_pd1/1
  Divide4_pd1/1 -> Out1/1

== system gm_uz_pmsm_model_9ph_21b_all_double/uz_pmsm_model_9ph/dq_model_9ph/Divide5 ==
  In1 : Inport
  In2 : Inport  Port=2
  Divide5 : Product  Inputs=**  OutDataTypeStr=double  SampleTime=1e-08
  Divide5_pd1 : Delay  DelayLength=6
  Out1 : Outport
  wires:
  In1/1 -> Divide5/1
  In2/1 -> Divide5/2
  Divide5/1 -> Divide5_pd1/1
  Divide5_pd1/1 -> Out1/1

== system gm_uz_pmsm_model_9ph_21b_all_double/uz_pmsm_model_9ph/dq_model_9ph/Divide6 ==
  In1 : Inport
  In2 : Inport  Port=2
  Divide6 : Product  Inputs=**  OutDataTypeStr=double  SampleTime=1e-08
  Divide6_pd1 : Delay  DelayLength=6
  Out1 : Outport
  wires:
  In1/1 -> Divide6/1
  In2/1 -> Divide6/2
  Divide6/1 -> Divide6_pd1/1
  Divide6_pd1/1 -> Out1/1

== system gm_uz_pmsm_model_9ph_21b_all_double/uz_pmsm_model_9ph/dq_model_9ph/Divide7 ==
  In1 : Inport
  In2 : Inport  Port=2
  Divide7 : Product  Inputs=**  OutDataTypeStr=double  SampleTime=1e-08
  Divide7_pd1 : Delay  DelayLength=6
  Out1 : Outport
  wires:
  In1/1 -> Divide7/1
  In2/1 -> Divide7/2
  Divide7/1 -> Divide7_pd1/1
  Divide7_pd1/1 -> Out1/1

== system gm_uz_pmsm_model_9ph_21b_all_double/uz_pmsm_model_9ph/dq_model_9ph/Divide8 ==
  In1 : Inport
  In2 : Inport  Port=2
  Divide8 : Product  Inputs=**  OutDataTypeStr=double  SampleTime=1e-08
  Divide8_pd1 : Delay  DelayLength=6
  Out1 : Outport
  wires:
  In1/1 -> Divide8/1
  In2/1 -> Divide8/2
  Divide8/1 -> Divide8_pd1/1
  Divide8_pd1/1 -> Out1/1

== system gm_uz_pmsm_model_9ph_21b_all_double/uz_pmsm_model_9ph/dq_model_9ph/Divide9 ==
  In1 : Inport
  In2 : Inport  Port=2
  Divide9 : Product  Inputs=**  OutDataTypeStr=double  SampleTime=1e-08
  Divide9_pd1 : Delay  DelayLength=6
  Out1 : Outport
  wires:
  In1/1 -> Divide9/1
  In2/1 -> Divide9/2
  Divide9/1 -> Divide9_pd1/1
  Divide9_pd1/1 -> Out1/1

== system gm_uz_pmsm_model_9ph_21b_all_double/uz_pmsm_model_9ph/dq_model_9ph/Factor ==
  In1 : Inport
  In2 : Inport  Port=2
  Factor : Product  Inputs=**  OutDataTypeStr=double  SampleTime=1e-08
  Factor_pd1 : Delay  DelayLength=6
  Out1 : Outport
  wires:
  In1/1 -> Factor/1
  In2/1 -> Factor/2
  Factor/1 -> Factor_pd1/1
  Factor_pd1/1 -> Out1/1

== system gm_uz_pmsm_model_9ph_21b_all_double/uz_pmsm_model_9ph/dq_model_9ph/Gain ==
  In1 : Inport
  In2 : Inport  Port=2
  Gain : Product  Inputs=**  OutDataTypeStr=double  SampleTime=1e-08
  Gain_pd1 : Delay  DelayLength=6
  Out1 : Outport
  wires:
  In1/1 -> Gain/1
  In2/1 -> Gain/2
  Gain/1 -> Gain_pd1/1
  Gain_pd1/1 -> Out1/1

== system gm_uz_pmsm_model_9ph_21b_all_double/uz_pmsm_model_9ph/dq_model_9ph/Gain1 ==
  In1 : Inport
  In2 : Inport  Port=2
  Gain1 : Product  Inputs=**  OutDataTypeStr=double  SampleTime=1e-08
  Gain1_pd1 : Delay  DelayLength=6
  Out1 : Outport
  wires:
  In1/1 -> Gain1/1
  In2/1 -> Gain1/2
  Gain1/1 -> Gain1_pd1/1
  Gain1_pd1/1 -> Out1/1

== system gm_uz_pmsm_model_9ph_21b_all_double/uz_pmsm_model_9ph/dq_model_9ph/Gain10 ==
  In1 : Inport
  In2 : Inport  Port=2
  Gain10 : Product  Inputs=**  OutDataTypeStr=double  SampleTime=1e-08
  Gain10_pd1 : Delay  DelayLength=6
  Out1 : Outport
  wires:
  In1/1 -> Gain10/1
  In2/1 -> Gain10/2
  Gain10/1 -> Gain10_pd1/1
  Gain10_pd1/1 -> Out1/1

== system gm_uz_pmsm_model_9ph_21b_all_double/uz_pmsm_model_9ph/dq_model_9ph/Gain2 ==
  In1 : Inport
  In2 : Inport  Port=2
  Gain2 : Product  Inputs=**  OutDataTypeStr=double  SampleTime=1e-08
  Gain2_pd1 : Delay  DelayLength=6
  Out1 : Outport
  wires:
  In1/1 -> Gain2/1
  In2/1 -> Gain2/2
  Gain2/1 -> Gain2_pd1/1
  Gain2_pd1/1 -> Out1/1

== system gm_uz_pmsm_model_9ph_21b_all_double/uz_pmsm_model_9ph/dq_model_9ph/Gain3 ==
  In1 : Inport
  In2 : Inport  Port=2
  Gain3 : Product  Inputs=**  OutDataTypeStr=double  SampleTime=1e-08
  Gain3_pd1 : Delay  DelayLength=6
  Out1 : Outport
  wires:
  In1/1 -> Gain3/1
  In2/1 -> Gain3/2
  Gain3/1 -> Gain3_pd1/1
  Gain3_pd1/1 -> Out1/1

== system gm_uz_pmsm_model_9ph_21b_all_double/uz_pmsm_model_9ph/dq_model_9ph/Gain4 ==
  In1 : Inport
  In2 : Inport  Port=2
  Gain4 : Product  Inputs=**  OutDataTypeStr=double  SampleTime=1e-08
  Gain4_pd1 : Delay  DelayLength=6
  Out1 : Outport
  wires:
  In1/1 -> Gain4/1
  In2/1 -> Gain4/2
  Gain4/1 -> Gain4_pd1/1
  Gain4_pd1/1 -> Out1/1

== system gm_uz_pmsm_model_9ph_21b_all_double/uz_pmsm_model_9ph/dq_model_9ph/Gain5 ==
  In1 : Inport
  In2 : Inport  Port=2
  Gain5 : Product  Inputs=**  OutDataTypeStr=double  SampleTime=1e-08
  Gain5_pd1 : Delay  DelayLength=6
  Out1 : Outport
  wires:
  In1/1 -> Gain5/1
  In2/1 -> Gain5/2
  Gain5/1 -> Gain5_pd1/1
  Gain5_pd1/1 -> Out1/1

== system gm_uz_pmsm_model_9ph_21b_all_double/uz_pmsm_model_9ph/dq_model_9ph/Gain6 ==
  In1 : Inport
  In2 : Inport  Port=2
  Gain6 : Product  Inputs=**  OutDataTypeStr=double  SampleTime=1e-08
  Gain6_pd1 : Delay  DelayLength=6
  Out1 : Outport
  wires:
  In1/1 -> Gain6/1
  In2/1 -> Gain6/2
  Gain6/1 -> Gain6_pd1/1
  Gain6_pd1/1 -> Out1/1

== system gm_uz_pmsm_model_9ph_21b_all_double/uz_pmsm_model_9ph/dq_model_9ph/Gain7 ==
  In1 : Inport
  In2 : Inport  Port=2
  Gain7 : Product  Inputs=**  OutDataTypeStr=double  SampleTime=1e-08
  Gain7_pd1 : Delay  DelayLength=6
  Out1 : Outport
  wires:
  In1/1 -> Gain7/1
  In2/1 -> Gain7/2
  Gain7/1 -> Gain7_pd1/1
  Gain7_pd1/1 -> Out1/1

== system gm_uz_pmsm_model_9ph_21b_all_double/uz_pmsm_model_9ph/dq_model_9ph/Gain8 ==
  In1 : Inport
  In2 : Inport  Port=2
  Gain8 : Product  Inputs=**  OutDataTypeStr=double  SampleTime=1e-08
  Gain8_pd1 : Delay  DelayLength=6
  Out1 : Outport
  wires:
  In1/1 -> Gain8/1
  In2/1 -> Gain8/2
  Gain8/1 -> Gain8_pd1/1
  Gain8_pd1/1 -> Out1/1

== system gm_uz_pmsm_model_9ph_21b_all_double/uz_pmsm_model_9ph/dq_model_9ph/Gain9 ==
  In1 : Inport
  In2 : Inport  Port=2
  Gain9 : Product  Inputs=**  OutDataTypeStr=double  SampleTime=1e-08
  Gain9_pd1 : Delay  DelayLength=6
  Out1 : Outport
  wires:
  In1/1 -> Gain9/1
  In2/1 -> Gain9/2
  Gain9/1 -> Gain9_pd1/1
  Gain9_pd1/1 -> Out1/1

== system gm_uz_pmsm_model_9ph_21b_all_double/uz_pmsm_model_9ph/dq_model_9ph/Product ==
  In1 : Inport
  In2 : Inport  Port=2
  Product : Product  Inputs=**  OutDataTypeStr=double  SampleTime=1e-08
  Product_pd1 : Delay  DelayLength=6
  Out1 : Outport
  wires:
  In1/1 -> Product/1
  In2/1 -> Product/2
  Product/1 -> Product_pd1/1
  Product_pd1/1 -> Out1/1

== system gm_uz_pmsm_model_9ph_21b_all_double/uz_pmsm_model_9ph/dq_model_9ph/Product1 ==
  In1 : Inport
  In2 : Inport  Port=2
  Product1 : Product  Inputs=**  OutDataTypeStr=double  SampleTime=1e-08
  Product1_pd1 : Delay  DelayLength=6
  Out1 : Outport
  wires:
  In1/1 -> Product1/1
  In2/1 -> Product1/2
  Product1/1 -> Product1_pd1/1
  Product1_pd1/1 -> Out1/1

== system gm_uz_pmsm_model_9ph_21b_all_double/uz_pmsm_model_9ph/dq_model_9ph/Product10 ==
  In1 : Inport
  In2 : Inport  Port=2
  Product10 : Product  Inputs=**  OutDataTypeStr=double  SampleTime=1e-08
  Product10_pd1 : Delay  DelayLength=6
  Out1 : Outport
  wires:
  In1/1 -> Product10/1
  In2/1 -> Product10/2
  Product10/1 -> Product10_pd1/1
  Product10_pd1/1 -> Out1/1

== system gm_uz_pmsm_model_9ph_21b_all_double/uz_pmsm_model_9ph/dq_model_9ph/Product11 ==
  In1 : Inport
  In2 : Inport  Port=2
  Product11 : Product  Inputs=**  OutDataTypeStr=double  SampleTime=1e-08
  Product11_pd1 : Delay  DelayLength=6
  Out1 : Outport
  wires:
  In1/1 -> Product11/1
  In2/1 -> Product11/2
  Product11/1 -> Product11_pd1/1
  Product11_pd1/1 -> Out1/1

== system gm_uz_pmsm_model_9ph_21b_all_double/uz_pmsm_model_9ph/dq_model_9ph/Product2 ==
  In1 : Inport
  In2 : Inport  Port=2
  Product2 : Product  Inputs=**  OutDataTypeStr=double  SampleTime=1e-08
  Product2_pd1 : Delay  DelayLength=6
  Out1 : Outport
  wires:
  In1/1 -> Product2/1
  In2/1 -> Product2/2
  Product2/1 -> Product2_pd1/1
  Product2_pd1/1 -> Out1/1

== system gm_uz_pmsm_model_9ph_21b_all_double/uz_pmsm_model_9ph/dq_model_9ph/Product3 ==
  In1 : Inport
  In2 : Inport  Port=2
  Product3 : Product  Inputs=**  OutDataTypeStr=double  SampleTime=1e-08
  Product3_pd1 : Delay  DelayLength=6
  Out1 : Outport
  wires:
  In1/1 -> Product3/1
  In2/1 -> Product3/2
  Product3/1 -> Product3_pd1/1
  Product3_pd1/1 -> Out1/1

== system gm_uz_pmsm_model_9ph_21b_all_double/uz_pmsm_model_9ph/dq_model_9ph/Product4 ==
  In1 : Inport
  In2 : Inport  Port=2
  Product4 : Product  Inputs=**  OutDataTypeStr=double  SampleTime=1e-08
  Product4_pd1 : Delay  DelayLength=6
  Out1 : Outport
  wires:
  In1/1 -> Product4/1
  In2/1 -> Product4/2
  Product4/1 -> Product4_pd1/1
  Product4_pd1/1 -> Out1/1

== system gm_uz_pmsm_model_9ph_21b_all_double/uz_pmsm_model_9ph/dq_model_9ph/Product5 ==
  In1 : Inport
  In2 : Inport  Port=2
  Product5 : Product  Inputs=**  OutDataTypeStr=double  SampleTime=1e-08
  Product5_pd1 : Delay  DelayLength=6
  Out1 : Outport
  wires:
  In1/1 -> Product5/1
  In2/1 -> Product5/2
  Product5/1 -> Product5_pd1/1
  Product5_pd1/1 -> Out1/1

== system gm_uz_pmsm_model_9ph_21b_all_double/uz_pmsm_model_9ph/dq_model_9ph/Product6 ==
  In1 : Inport
  In2 : Inport  Port=2
  Product6 : Product  Inputs=**  OutDataTypeStr=double  SampleTime=1e-08
  Product6_pd1 : Delay  DelayLength=6
  Out1 : Outport
  wires:
  In1/1 -> Product6/1
  In2/1 -> Product6/2
  Product6/1 -> Product6_pd1/1
  Product6_pd1/1 -> Out1/1

== system gm_uz_pmsm_model_9ph_21b_all_double/uz_pmsm_model_9ph/dq_model_9ph/Product7 ==
  In1 : Inport
  In2 : Inport  Port=2
  Product7 : Product  Inputs=**  OutDataTypeStr=double  SampleTime=1e-08
  Product7_pd1 : Delay  DelayLength=6
  Out1 : Outport
  wires:
  In1/1 -> Product7/1
  In2/1 -> Product7/2
  Product7/1 -> Product7_pd1/1
  Product7_pd1/1 -> Out1/1

== system gm_uz_pmsm_model_9ph_21b_all_double/uz_pmsm_model_9ph/dq_model_9ph/Product8 ==
  In1 : Inport
  In2 : Inport  Port=2
  Product8 : Product  Inputs=**  OutDataTypeStr=double  SampleTime=1e-08
  Product8_pd1 : Delay  DelayLength=6
  Out1 : Outport
  wires:
  In1/1 -> Product8/1
  In2/1 -> Product8/2
  Product8/1 -> Product8_pd1/1
  Product8_pd1/1 -> Out1/1

== system gm_uz_pmsm_model_9ph_21b_all_double/uz_pmsm_model_9ph/dq_model_9ph/Product9 ==
  In1 : Inport
  In2 : Inport  Port=2
  Product9 : Product  Inputs=**  OutDataTypeStr=double  SampleTime=1e-08
  Product9_pd1 : Delay  DelayLength=6
  Out1 : Outport
  wires:
  In1/1 -> Product9/1
  In2/1 -> Product9/2
  Product9/1 -> Product9_pd1/1
  Product9_pd1/1 -> Out1/1

== system gm_uz_pmsm_model_9ph_21b_all_double/uz_pmsm_model_9ph/dq_model_9ph/Sum ==
  In1 : Inport
  In2 : Inport  Port=2
  Sum : Sum  OutDataTypeStr=double  SampleTime=1e-08
  Sum_pd1 : Delay  DelayLength=6
  Out1 : Outport
  wires:
  In1/1 -> Sum/1
  In2/1 -> Sum/2
  Sum/1 -> Sum_pd1/1
  Sum_pd1/1 -> Out1/1

== system gm_uz_pmsm_model_9ph_21b_all_double/uz_pmsm_model_9ph/dq_model_9ph/Sum1 ==
  In1 : Inport
  In2 : Inport  Port=2
  Sum1 : Sum  Inputs=+-  OutDataTypeStr=double  SampleTime=1e-08
  Sum1_pd1 : Delay  DelayLength=6
  Out1 : Outport
  wires:
  In1/1 -> Sum1/1
  In2/1 -> Sum1/2
  Sum1/1 -> Sum1_pd1/1
  Sum1_pd1/1 -> Out1/1

== system gm_uz_pmsm_model_9ph_21b_all_double/uz_pmsm_model_9ph/dq_model_9ph/Sum11 ==
  In1 : Inport
  In2 : Inport  Port=2
  Sum11 : Sum  OutDataTypeStr=double  SampleTime=1e-08
  Sum11_pd1 : Delay  DelayLength=6
  Out1 : Outport
  wires:
  In1/1 -> Sum11/1
  In2/1 -> Sum11/2
  Sum11/1 -> Sum11_pd1/1
  Sum11_pd1/1 -> Out1/1

== system gm_uz_pmsm_model_9ph_21b_all_double/uz_pmsm_model_9ph/dq_model_9ph/Sum1_stage2 ==
  In1 : Inport
  In2 : Inport  Port=2
  Sum1_stage2 : Sum  Inputs=+-  OutDataTypeStr=double  SampleTime=1e-08
  Sum1_stage2_pd1 : Delay  DelayLength=6
  Out1 : Outport
  wires:
  In1/1 -> Sum1_stage2/1
  In2/1 -> Sum1_stage2/2
  Sum1_stage2/1 -> Sum1_stage2_pd1/1
  Sum1_stage2_pd1/1 -> Out1/1

== system gm_uz_pmsm_model_9ph_21b_all_double/uz_pmsm_model_9ph/dq_model_9ph/Sum1_stage3 ==
  In1 : Inport
  In2 : Inport  Port=2
  Sum1_stage3 : Sum  Inputs=+-  OutDataTypeStr=double  SampleTime=1e-08
  Sum1_stage3_pd1 : Delay  DelayLength=6
  Out1 : Outport
  wires:
  In1/1 -> Sum1_stage3/1
  In2/1 -> Sum1_stage3/2
  Sum1_stage3/1 -> Sum1_stage3_pd1/1
  Sum1_stage3_pd1/1 -> Out1/1

== system gm_uz_pmsm_model_9ph_21b_all_double/uz_pmsm_model_9ph/dq_model_9ph/Sum2 ==
  In1 : Inport
  In2 : Inport  Port=2
  Sum2 : Sum  OutDataTypeStr=double  SampleTime=1e-08
  Sum2_pd1 : Delay  DelayLength=6
  Out1 : Outport
  wires:
  In1/1 -> Sum2/1
  In2/1 -> Sum2/2
  Sum2/1 -> Sum2_pd1/1
  Sum2_pd1/1 -> Out1/1
